simulink model "ModelMotS_dq"  (R2018b)
settings: Solver=ode45  StartTime=0.0  StopTime=1  MaxStep=1e-4  RelTol=1e-4  EnableMultiTasking=on
values from neighbouring files (symbols this model uses):
  J = 0.045    [gen_sim.m]    (also in gen_sim_new_data_december.m)
  Lfr = 0.007    [gen_sim.m]    (also in gen_sim_new_data_december.m)
  Lfs = 0.007    [gen_sim.m]    (also in gen_sim_new_data_december.m)
  Lmt = 0.210    (= 0.21)    [gen_sim.m]    (also in gen_sim_new_data_december.m)
  Lr = 0.160    (= 0.16)    [gen_sim.m]    (also in gen_sim_new_data_december.m)
  np = 2    [gen_sim.m]    (also in gen_sim_new_data_december.m)
  P1 = 0.7    [gen_sim.m]    (also in gen_sim_new_data_december.m)
  P2 = 1.5    [gen_sim.m]    (also in gen_sim_new_data_december.m)
  Prinit = [ 0 ; 0 ]    [gen_sim.m]    (also in gen_sim_new_data_december.m)
  Psdnom = 0.95    [gen_sim.m]    (also in gen_sim_new_data_december.m)
  Psinit = [ 0 ; 0 ]    [gen_sim.m]    (also in gen_sim_new_data_december.m)
  Rr = 0.9    [gen_sim.m]    (also in gen_sim_new_data_december.m)
  Rs = 1.5    [gen_sim.m]    (also in gen_sim_new_data_december.m)
  tauL = 25    [gen_sim.m]    (also in gen_sim_new_data_december.m)
  thrinit = 0    [gen_sim.m]    (also in gen_sim_new_data_december.m)
  Ts = 0.000250    (= 0.00025)    [gen_sim.m]    (also in gen_sim_new_data_december.m)
  Ulim = 415*sqrt(2/3)    [gen_sim.m]    (also in gen_sim_new_data_december.m)
  Uo = 15    [gen_sim.m]    (also in gen_sim_new_data_december.m)
  wL = 2*pi*0    (= 0)    [gen_sim.m]    (also in gen_sim_new_data_december.m)
  wrinit = 2*pi*0    (= 0)    [gen_sim.m]    (also in gen_sim_new_data_december.m)
libraries: simulink x5
(part 2 of 2)

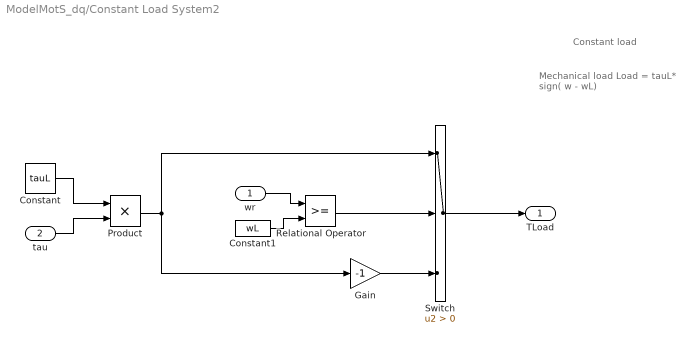
== system ModelMotS_dq/Constant Load System2 ==
  note: Constant load
  note: Mechanical load
      |  Load = tauL* sign( w - wL)
  wr : Inport
  tau : Inport  Port=2
  Constant : Constant  Value=tauL
  Constant1 : Constant  Value=wL
  Gain : Gain  Gain=-1
  Product : Product
  Relational Operator : RelationalOperator  OutDataTypeStr=boolean  ZeroCross=off  RndMeth=Nearest
  Switch : Switch  Criteria=u2 > Threshold
  TLoad : Outport
  wires:
  Gain/1 -> Switch/3
  Switch/1 -> TLoad/1
  Product/1 -> Gain/1, Switch/1
  Relational Operator/1 -> Switch/2
  wr/1 -> Relational Operator/1
  Constant1/1 -> Relational Operator/2
  Constant/1 -> Product/1
  tau/1 -> Product/2

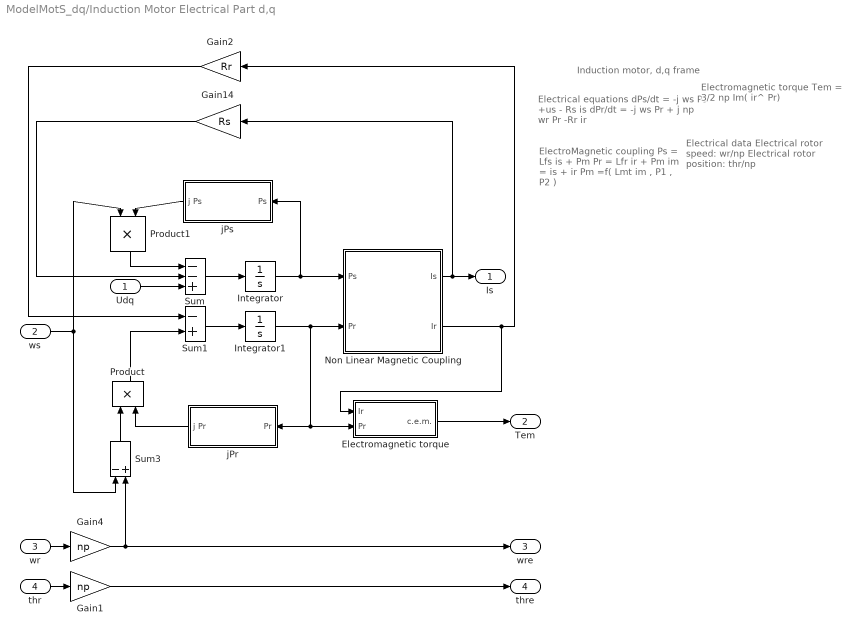
== system ModelMotS_dq/Induction Motor Electrical Part d,q ==
  note: Electrical equations
      | dPs/dt =  -j ws Ps +us - Rs is
      | dPr/dt = -j ws Pr + j np wr Pr -Rr ir
  note: Electromagnetic torque
      | Tem = 3/2 np Im( ir^ Pr)
  note: Induction motor, d,q frame
  note: Electrical data
      | Electrical rotor speed: wr/np
      | Electrical rotor position: thr/np
  note: ElectroMagnetic coupling
      | Ps  = Lfs is + Pm
      | Pr  = Lfr ir + Pm
      |
      | im = is + ir
      | Pm =f( Lmt im , P1 , P2 )
  Udq : Inport
  ws : Inport  Port=2
  wr : Inport  Port=3
  thr : Inport  Port=4
  Electromagnetic torque : Subsystem
  Gain1 : Gain  Gain=np  SaturateOnIntegerOverflow=on  OutDataTypeStr=Inherit: Same as input  ParamDataTypeStr=Inherit: Same as input
  Gain14 : Gain  Gain=Rs  SaturateOnIntegerOverflow=on  OutDataTypeStr=Inherit: Same as input  ParamDataTypeStr=Inherit: Same as input
  Gain2 : Gain  Gain=Rr  SaturateOnIntegerOverflow=on  OutDataTypeStr=Inherit: Same as input  ParamDataTypeStr=Inherit: Same as input
  Gain4 : Gain  Gain=np  SaturateOnIntegerOverflow=on  OutDataTypeStr=Inherit: Same as input  ParamDataTypeStr=Inherit: Same as input
  Integrator : Integrator  InitialCondition=Psinit
  Integrator1 : Integrator  InitialCondition=Prinit
  Non Linear Magnetic Coupling : Subsystem
  Product : Product  SaturateOnIntegerOverflow=on  RndMeth=Zero  InputSameDT=on  OutDataTypeStr=Inherit: Same as first input
  Product1 : Product  SaturateOnIntegerOverflow=on  RndMeth=Zero  InputSameDT=on  OutDataTypeStr=Inherit: Same as first input
  Sum : Sum  Inputs=--+  SaturateOnIntegerOverflow=on  InputSameDT=on  OutDataTypeStr=Inherit: Same as first input
  Sum1 : Sum  Inputs=-+  SaturateOnIntegerOverflow=on  InputSameDT=on  OutDataTypeStr=Inherit: Same as first input
  Sum3 : Sum  Inputs=-+  SaturateOnIntegerOverflow=on  InputSameDT=on  OutDataTypeStr=Inherit: Same as first input
  jPr : Subsystem
  jPs : Subsystem
  Is : Outport
  Tem : Outport  Port=2
  wre : Outport  Port=3
  thre : Outport  Port=4
  wires:
  Integrator1/1 -> Non Linear Magnetic Coupling/2(Pr), Electromagnetic torque/2(Pr), jPr/1(Pr)
  Electromagnetic torque/1(c.e.m.) -> Tem/1
  Non Linear Magnetic Coupling/2(Ir) -> Electromagnetic torque/1(Ir), Gain2/1
  Product/1 -> Sum1/2
  jPr/1(j Pr) -> Product/2
  Gain2/1 -> Sum1/1
  Sum1/1 -> Integrator1/1
  Non Linear Magnetic Coupling/1(Is) -> Is/1, Gain14/1
  Sum/1 -> Integrator/1
  Udq/1 -> Sum/3
  Gain14/1 -> Sum/2
  jPs/1(j Ps) -> Product1/2
  Product1/1 -> Sum/1
  Integrator/1 -> Non Linear Magnetic Coupling/1(Ps), jPs/1(Ps)
  Sum3/1 -> Product/1
  Gain4/1 -> wre/1, Sum3/2
  ws/1 -> Product1/1, Sum3/1
  wr/1 -> Gain4/1
  thr/1 -> Gain1/1
  Gain1/1 -> thre/1

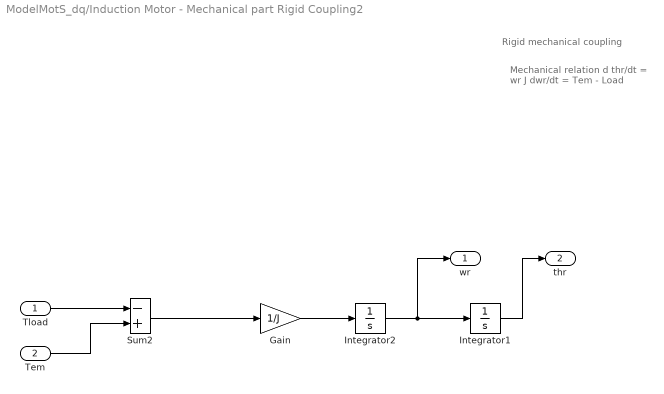
== system ModelMotS_dq/Induction Motor - Mechanical part Rigid Coupling2 ==
  note: Rigid mechanical coupling
  note: Mechanical relation
      | d thr/dt = wr
      | J dwr/dt = Tem - Load
  Tload : Inport
  Tem : Inport  Port=2
  Gain : Gain  Gain=1/J  SaturateOnIntegerOverflow=on  OutDataTypeStr=Inherit: Same as input  ParamDataTypeStr=Inherit: Same as input
  Integrator1 : Integrator  InitialCondition=thrinit
  Integrator2 : Integrator  InitialCondition=wrinit
  Sum2 : Sum  Inputs=-+  SaturateOnIntegerOverflow=on  InputSameDT=on  OutDataTypeStr=Inherit: Same as first input
  wr : Outport
  thr : Outport  Port=2
  wires:
  Integrator1/1 -> thr/1
  Integrator2/1 -> wr/1, Integrator1/1
  Tem/1 -> Sum2/2
  Tload/1 -> Sum2/1
  Gain/1 -> Integrator2/1
  Sum2/1 -> Gain/1

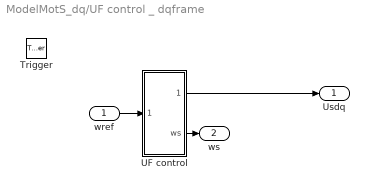
== system ModelMotS_dq/UF control _ dqframe ==
  wref : Inport
  Trigger : TriggerPort  VariantControl=(inherit)  PortDimensions=1
  UF control : Subsystem
  Usdq : Outport
  ws : Outport  Port=2
  wires:
  UF control/1(Udq) -> Usdq/1
  wref/1 -> UF control/1(wref)
  UF control/2(ws) -> ws/1

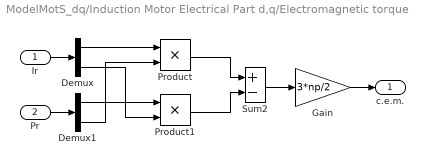
== system ModelMotS_dq/Induction Motor Electrical Part d,q/Electromagnetic torque ==
  Ir : Inport
  Pr : Inport  Port=2
  Demux : Demux  Outputs=2
  Demux1 : Demux  Outputs=2
  Gain : Gain  Gain=3*np/2  SaturateOnIntegerOverflow=on  OutDataTypeStr=Inherit: Same as input  ParamDataTypeStr=Inherit: Same as input
  Product : Product  SaturateOnIntegerOverflow=on  RndMeth=Zero  InputSameDT=on  OutDataTypeStr=Inherit: Same as first input
  Product1 : Product  SaturateOnIntegerOverflow=on  RndMeth=Zero  InputSameDT=on  OutDataTypeStr=Inherit: Same as first input
  Sum2 : Sum  Inputs=+-  SaturateOnIntegerOverflow=on  InputSameDT=on  OutDataTypeStr=Inherit: Same as first input
  c.e.m. : Outport
  wires:
  Pr/1 -> Demux1/1
  Gain/1 -> c.e.m./1
  Ir/1 -> Demux/1
  Demux/2 -> Product1/2
  Demux1/1 -> Product1/1
  Demux1/2 -> Product/2
  Demux/1 -> Product/1
  Sum2/1 -> Gain/1
  Product1/1 -> Sum2/2
  Product/1 -> Sum2/1

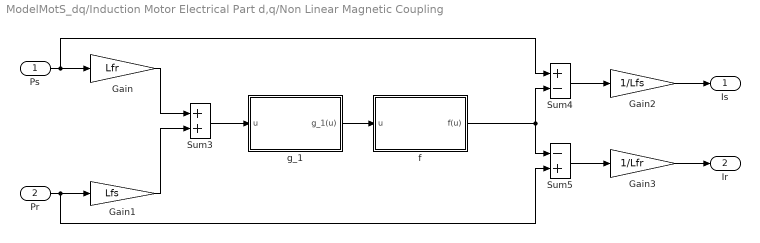
== system ModelMotS_dq/Induction Motor Electrical Part d,q/Non Linear Magnetic Coupling ==
  Ps : Inport
  Pr : Inport  Port=2
  Gain : Gain  Gain=Lfr  SaturateOnIntegerOverflow=on  OutDataTypeStr=Inherit: Same as input  ParamDataTypeStr=Inherit: Same as input
  Gain1 : Gain  Gain=Lfs  SaturateOnIntegerOverflow=on  OutDataTypeStr=Inherit: Same as input  ParamDataTypeStr=Inherit: Same as input
  Gain2 : Gain  Gain=1/Lfs  SaturateOnIntegerOverflow=on  OutDataTypeStr=Inherit: Same as input  ParamDataTypeStr=Inherit: Same as input
  Gain3 : Gain  Gain=1/Lfr  SaturateOnIntegerOverflow=on  OutDataTypeStr=Inherit: Same as input  ParamDataTypeStr=Inherit: Same as input
  Sum3 : Sum  SaturateOnIntegerOverflow=on  InputSameDT=on  OutDataTypeStr=Inherit: Same as first input
  Sum4 : Sum  Inputs=+-  SaturateOnIntegerOverflow=on  InputSameDT=on  OutDataTypeStr=Inherit: Same as first input
  Sum5 : Sum  Inputs=-+  SaturateOnIntegerOverflow=on  InputSameDT=on  OutDataTypeStr=Inherit: Same as first input
  f : Subsystem
  g_1 : Subsystem
  Is : Outport
  Ir : Outport  Port=2
  wires:
  Gain2/1 -> Is/1
  Gain3/1 -> Ir/1
  Sum5/1 -> Gain3/1
  Sum4/1 -> Gain2/1
  Pr/1 -> Sum5/2, Gain1/1
  Ps/1 -> Sum4/1, Gain/1
  f/1(f(u)) -> Sum4/2, Sum5/1
  g_1/1(g_1(u)) -> f/1(u)
  Sum3/1 -> g_1/1(u)
  Gain1/1 -> Sum3/2
  Gain/1 -> Sum3/1

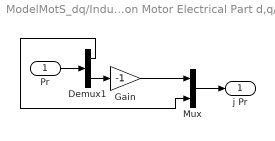
== system ModelMotS_dq/Induction Motor Electrical Part d,q/jPr ==
  Pr : Inport
  Demux1 : Demux  Outputs=2
  Gain : Gain  Gain=-1  SaturateOnIntegerOverflow=on  OutDataTypeStr=Inherit: Same as input  ParamDataTypeStr=Inherit: Same as input
  Mux : Mux  Inputs=2
  j Pr : Outport
  wires:
  Mux/1 -> j Pr/1
  Gain/1 -> Mux/1
  Demux1/2 -> Gain/1
  Demux1/1 -> Mux/2
  Pr/1 -> Demux1/1

== system ModelMotS_dq/Induction Motor Electrical Part d,q/jPs ==
  Ps : Inport
  Demux1 : Demux  Outputs=2
  Gain : Gain  Gain=-1  SaturateOnIntegerOverflow=on  OutDataTypeStr=Inherit: Same as input  ParamDataTypeStr=Inherit: Same as input
  Mux : Mux  Inputs=2
  j Ps : Outport
  wires:
  Ps/1 -> Demux1/1
  Demux1/1 -> Mux/2
  Demux1/2 -> Gain/1
  Gain/1 -> Mux/1
  Mux/1 -> j Ps/1

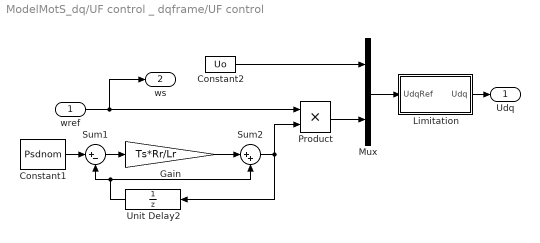
== system ModelMotS_dq/UF control _ dqframe/UF control ==
  wref : Inport
  Constant1 : Constant  Value=Psdnom
  Constant2 : Constant  Value=Uo
  Gain : Gain  Gain=Ts*Rr/Lr
  Limitation : Subsystem
  Mux : Mux  Inputs=2
  Product : Product
  Sum1 : Sum  Inputs=|+-
  Sum2 : Sum  Inputs=|++
  Unit Delay2 : UnitDelay  SampleTime=-1
  Udq : Outport
  ws : Outport  Port=2
  wires:
  Mux/1 -> Limitation/1(UdqRef)
  Sum2/1 -> Product/2, Unit Delay2/1
  wref/1 -> ws/1, Product/1
  Product/1 -> Mux/2
  Constant2/1 -> Mux/1
  Constant1/1 -> Sum1/1
  Unit Delay2/1 -> Sum2/2, Sum1/2
  Sum1/1 -> Gain/1
  Gain/1 -> Sum2/1
  Limitation/1(Udq) -> Udq/1

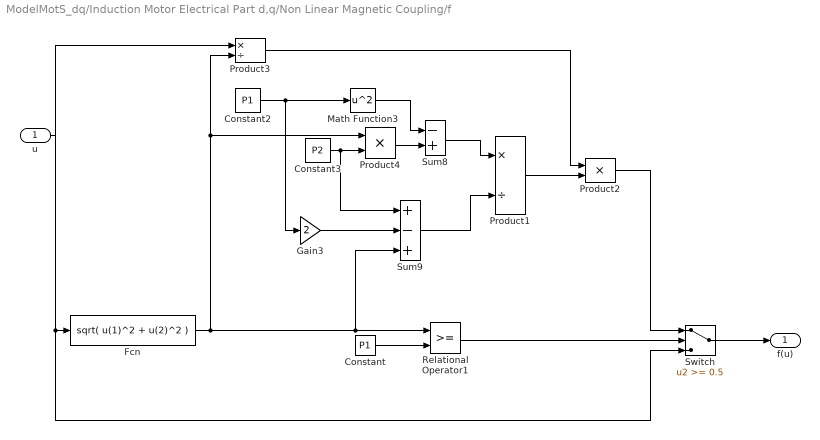
== system ModelMotS_dq/Induction Motor Electrical Part d,q/Non Linear Magnetic Coupling/f ==
  u : Inport
  Constant : Constant  Value=P1
  Constant2 : Constant  Value=P1
  Constant3 : Constant  Value=P2
  Fcn : Fcn  Expr=sqrt( u(1)^2 + u(2)^2 )
  Gain3 : Gain  Gain=2  SaturateOnIntegerOverflow=on  OutDataTypeStr=Inherit: Same as input  ParamDataTypeStr=Inherit: Same as input
  Math Function3 : Math  Operator=square  SaturateOnIntegerOverflow=on
  Product1 : Product  Inputs=*/  SaturateOnIntegerOverflow=on  RndMeth=Zero  InputSameDT=on  OutDataTypeStr=Inherit: Same as first input
  Product2 : Product  SaturateOnIntegerOverflow=on  RndMeth=Zero  InputSameDT=on  OutDataTypeStr=Inherit: Same as first input
  Product3 : Product  Inputs=*/  SaturateOnIntegerOverflow=on  RndMeth=Zero  InputSameDT=on  OutDataTypeStr=Inherit: Same as first input
  Product4 : Product  SaturateOnIntegerOverflow=on  RndMeth=Zero  InputSameDT=on  OutDataTypeStr=Inherit: Same as first input
  Relational Operator1 : RelationalOperator  RndMeth=Nearest  InputSameDT=on
  Sum8 : Sum  Inputs=-+  SaturateOnIntegerOverflow=on  InputSameDT=on  OutDataTypeStr=Inherit: Same as first input
  Sum9 : Sum  Inputs=+-+  SaturateOnIntegerOverflow=on  InputSameDT=on  OutDataTypeStr=Inherit: Same as first input
  Switch : Switch  Threshold=0.5  SaturateOnIntegerOverflow=on  InputSameDT=on
  f(u) : Outport  InitialOutput=0
  wires:
  Fcn/1 -> Sum9/3, Relational Operator1/1, Product4/1, Product3/2
  Switch/1 -> f(u)/1
  Sum8/1 -> Product1/1
  Sum9/1 -> Product1/2
  Constant2/1 -> Gain3/1, Math Function3/1
  Gain3/1 -> Sum9/2
  Constant3/1 -> Sum9/1, Product4/2
  Math Function3/1 -> Sum8/1
  Product4/1 -> Sum8/2
  Product1/1 -> Product2/2
  Product3/1 -> Product2/1
  u/1 -> Switch/3, Fcn/1, Product3/1
  Relational Operator1/1 -> Switch/2
  Constant/1 -> Relational Operator1/2
  Product2/1 -> Switch/1

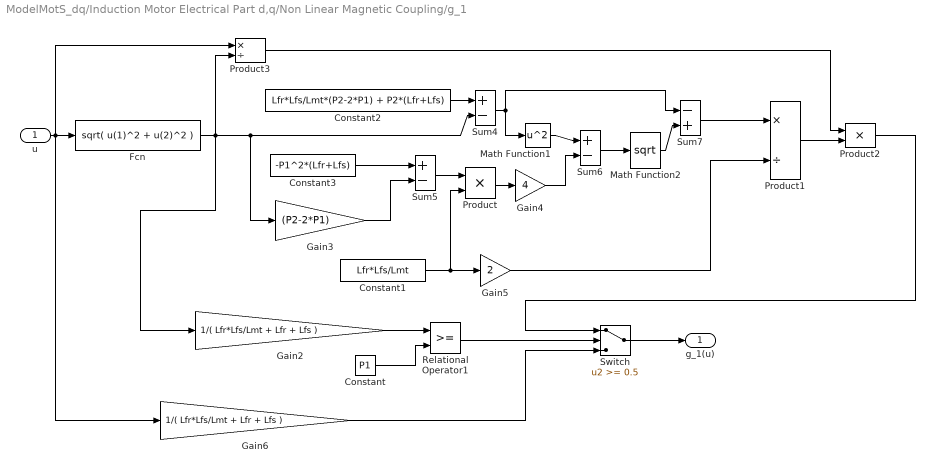
== system ModelMotS_dq/Induction Motor Electrical Part d,q/Non Linear Magnetic Coupling/g_1 ==
  u : Inport
  Constant : Constant  Value=P1
  Constant1 : Constant  Value=Lfr*Lfs/Lmt
  Constant2 : Constant  Value=Lfr*Lfs/Lmt*(P2-2*P1) + P2*(Lfr+Lfs)
  Constant3 : Constant  Value=-P1^2*(Lfr+Lfs)
  Fcn : Fcn  Expr=sqrt( u(1)^2 + u(2)^2 )
  Gain2 : Gain  Gain=1/( Lfr*Lfs/Lmt + Lfr + Lfs )  SaturateOnIntegerOverflow=on  OutDataTypeStr=Inherit: Same as input  ParamDataTypeStr=Inherit: Same as input
  Gain3 : Gain  Gain=(P2-2*P1)  SaturateOnIntegerOverflow=on  OutDataTypeStr=Inherit: Same as input  ParamDataTypeStr=Inherit: Same as input
  Gain4 : Gain  Gain=4  SaturateOnIntegerOverflow=on  OutDataTypeStr=Inherit: Same as input  ParamDataTypeStr=Inherit: Same as input
  Gain5 : Gain  Gain=2  SaturateOnIntegerOverflow=on  OutDataTypeStr=Inherit: Same as input  ParamDataTypeStr=Inherit: Same as input
  Gain6 : Gain  Gain=1/( Lfr*Lfs/Lmt + Lfr + Lfs )  SaturateOnIntegerOverflow=on  OutDataTypeStr=Inherit: Same as input  ParamDataTypeStr=Inherit: Same as input
  Math Function1 : Math  Operator=square  SaturateOnIntegerOverflow=on
  Math Function2 : Math  Operator=sqrt  SaturateOnIntegerOverflow=on
  Product : Product  SaturateOnIntegerOverflow=on  RndMeth=Zero  InputSameDT=on  OutDataTypeStr=Inherit: Same as first input
  Product1 : Product  Inputs=*/  SaturateOnIntegerOverflow=on  RndMeth=Zero  InputSameDT=on  OutDataTypeStr=Inherit: Same as first input
  Product2 : Product  SaturateOnIntegerOverflow=on  RndMeth=Zero  InputSameDT=on  OutDataTypeStr=Inherit: Same as first input
  Product3 : Product  Inputs=*/  SaturateOnIntegerOverflow=on  RndMeth=Zero  InputSameDT=on  OutDataTypeStr=Inherit: Same as first input
  Relational Operator1 : RelationalOperator  RndMeth=Nearest  InputSameDT=on
  Sum4 : Sum  Inputs=+-  SaturateOnIntegerOverflow=on  InputSameDT=on  OutDataTypeStr=Inherit: Same as first input
  Sum5 : Sum  Inputs=+-  SaturateOnIntegerOverflow=on  InputSameDT=on  OutDataTypeStr=Inherit: Same as first input
  Sum6 : Sum  Inputs=+-  SaturateOnIntegerOverflow=on  InputSameDT=on  OutDataTypeStr=Inherit: Same as first input
  Sum7 : Sum  Inputs=-+  SaturateOnIntegerOverflow=on  InputSameDT=on  OutDataTypeStr=Inherit: Same as first input
  Switch : Switch  Threshold=0.5  SaturateOnIntegerOverflow=on  InputSameDT=on
  g_1(u) : Outport  InitialOutput=0
  wires:
  Switch/1 -> g_1(u)/1
  Gain6/1 -> Switch/3
  Product2/1 -> Switch/1
  Constant/1 -> Relational Operator1/2
  Gain2/1 -> Relational Operator1/1
  Relational Operator1/1 -> Switch/2
  u/1 -> Gain6/1, Product3/1, Fcn/1
  Product3/1 -> Product2/1
  Fcn/1 -> Gain2/1, Product3/2, Gain3/1, Sum4/2
  Constant1/1 -> Gain5/1, Product/2
  Sum5/1 -> Product/1
  Product/1 -> Gain4/1
  Product1/1 -> Product2/2
  Gain5/1 -> Product1/2
  Sum7/1 -> Product1/1
  Gain3/1 -> Sum5/2
  Constant3/1 -> Sum5/1
  Sum4/1 -> Sum7/1, Math Function1/1
  Math Function2/1 -> Sum7/2
  Sum6/1 -> Math Function2/1
  Math Function1/1 -> Sum6/1
  Constant2/1 -> Sum4/1
  Gain4/1 -> Sum6/2

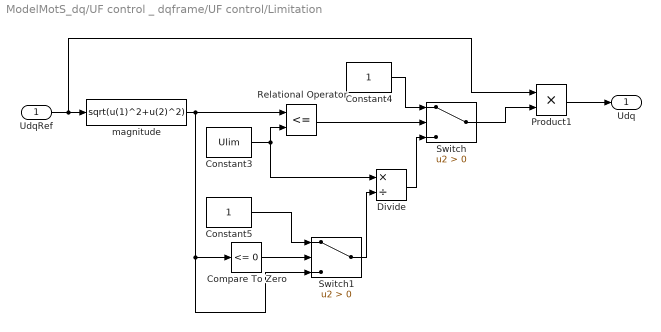
== system ModelMotS_dq/UF control _ dqframe/UF control/Limitation ==
  UdqRef : Inport
  Compare To Zero : simulink/Logic and Bit Operations/Compare To Zero  relop=<=  OutDataTypeStr=boolean
  Constant3 : Constant  Value=Ulim
  Constant4 : Constant
  Constant5 : Constant
  Divide : Product  Inputs=*/
  Product1 : Product
  Relational Operator : RelationalOperator  Operator=<=  OutDataTypeStr=boolean  RndMeth=Nearest
  Switch : Switch  Criteria=u2 > Threshold
  Switch1 : Switch  Criteria=u2 > Threshold
  magnitude : Fcn  Expr=sqrt(u(1)^2+u(2)^2)
  Udq : Outport
  wires:
  Constant3/1 -> Divide/1, Relational Operator/2
  Compare To Zero/1 -> Switch1/2
  Switch1/1 -> Divide/2
  Constant4/1 -> Switch/1
  UdqRef/1 -> Product1/1, magnitude/1
  Divide/1 -> Switch/3
  Constant5/1 -> Switch1/1
  Switch/1 -> Product1/2
  Product1/1 -> Udq/1
  Relational Operator/1 -> Switch/2
  magnitude/1 -> Compare To Zero/1, Switch1/3, Relational Operator/1
